simulink model "STDiscovery"  (R2017b)
settings: Solver=FixedStepAuto  StartTime=0.0  StopTime=0.01  FixedStep=Abtastzeit  RelTol=1e-3
PreLoadFcn:
  | waijung.modelPreload; % Required for working with Waijung Blockset. Do not remove.
model workspace (MAT data in the model file):
  Abtastzeit = 0.01
  Servo_IN_min = 0.894
  SimulationDutyCycle = 27
undefined symbols (not defined in the file): HSEOSC, Link, LQFP176, ST, Statusbits, Steuerbits, STM32F417IG
libraries: simulink x17, stm32f4_io_lib x16, simulink_extras x8, stm32f4_adc_lib x7, powerlib_meascontrol x4, stm32f4_device_config_lib x1
(part 2 of 4)

== system STDiscovery/MomentangeschwindigkeitEinlesen ==
  note: Umrechnung Hz nach m/s
  Data Store Write : DataStoreWrite  DataStoreName=MomentanGeschwindigkeit_MeterProSekunde
  Fernbediehnung Motor : S-Function  FunctionName=stm32f4_pwm_capture  Parameters=conf,inputporttype,inputportwidth,outputporttype,outputportwidth,optionstring,sampletime,blockid  SFunctionDeploymentMode=off  EnableBusSupport=off  mask(stm32f4_pwm_capture){conf=Capture, timer=3, lasttimer=3, pin=C7, pintype=Pull Up, edge=Rising, datatype=single, portpinstr=0, sampletime=Abtastzeit, blockid=MomentangeschwindigkeitEinlesenFernbediehnungMotor, inputporttype=[], inputportwidth=[], inputportlabel={}, outputporttype=[3 1 1 1], outputportwidth=[], outputportlabel={'READY','+Width (sec)','+Duty (%)','Frequency (Hz)'}, compat=0, optionstring=["3","1","C","7","2","16","Rising","UP","float"]}
      mask prompts: conf "Configuration"; lasttimer "Last Timer"; pin "Capture Pin"; pintype "Capture Pin Type (Pull-Up/Pull-Down)"; edge "Capture Edge"; datatype "Output data type"; portpinstr "Port Pin String"; sampletime "Sample time (sec)"; blockid "Block ID"; inputporttype "Input Port Type"; inputportwidth "Input Port Width"; inputportlabel "Input Port Label"; outputporttype "Output Port Type"; outputportwidth "Output Port Width"; outputportlabel "Output port label"; compat "Compatibility (Reserved for future use)"; optionstring "String(s) to be passed to TLC"
      mask help:
      | Capture Edge:
      |  Rising - PWM period start from rising edge of pulse N to rising edge of pulse N+1
      |  Falling - PWM period start from falling edge of pulse N to falling edge of pulse N+1
      | Capture data type:
      |  Capture data type, selectable to double or single.
      |
      | Output:
      |  READY - indicate the status of capture, a non-zero value indicate data is ready.
      |  +Width - positive pulse width, in unit of second.
      |  +Duty - positive duty cycle, 0 to 100%
      |  Frequency - signal frequency in unit of Hz
      |
      | Note: caprure period should not longer than 1 second (Maximum limit is 3 seconds)
      mask init:
      | stm32f4_pwm_capture_callback('init');
      mask Help: web(fullfile(waijungdocroot,'stm32f4_pwm_capture.htm'), '-browser')
      mask TypeOptions conf: Capture
      mask Callback conf: stm32f4_pwm_capture_callback('conf');
      mask TypeOptions timer: 1 | 2 | 3 | 4 | 5 | 8
      mask Callback timer: stm32f4_pwm_capture_callback('timer');
      mask TypeOptions pin: Not used | A6 | B4 | C6 | A7 | B5 | C7 | B0 | C8 | B1 | C9
      mask TypeOptions pintype: None | Pull Up | Pull Down
      mask TypeOptions edge: Rising | Falling
      mask TypeOptions datatype: double | single
      mask Callback sampletime: stm32f4_pwm_capture_callback('sampletime');
      mask Callback blockid: stm32f4_pwm_capture_callback('blockid');
      mask Display: text(0.05, 0.5, 'Timer: 3 (16 bit)\nInput Pin: C7\nEdge: Rising\nTs (sec): -1','ver','middle','hor','left'); port_label('output', 1,'READY'); port_label('output', 2,'+Width (sec)'); port_label('output', 3,'+Duty (%)'); port_label('output', 4,'Frequency (Hz)');
  MATLAB Function : MATLAB Function  TreatAsAtomicUnit=on
  Saturation : Saturate  UpperLimit=10  LowerLimit=0
  Terminator : Terminator
  Terminator1 : Terminator
  Terminator2 : Terminator
  wires:
  MATLAB Function/1(y) -> Saturation/1
  Saturation/1 -> Data Store Write/1
  Fernbediehnung Motor/4 -> MATLAB Function/1(x)
  Fernbediehnung Motor/1 -> Terminator/1
  Fernbediehnung Motor/2 -> Terminator1/1
  Fernbediehnung Motor/3 -> Terminator2/1

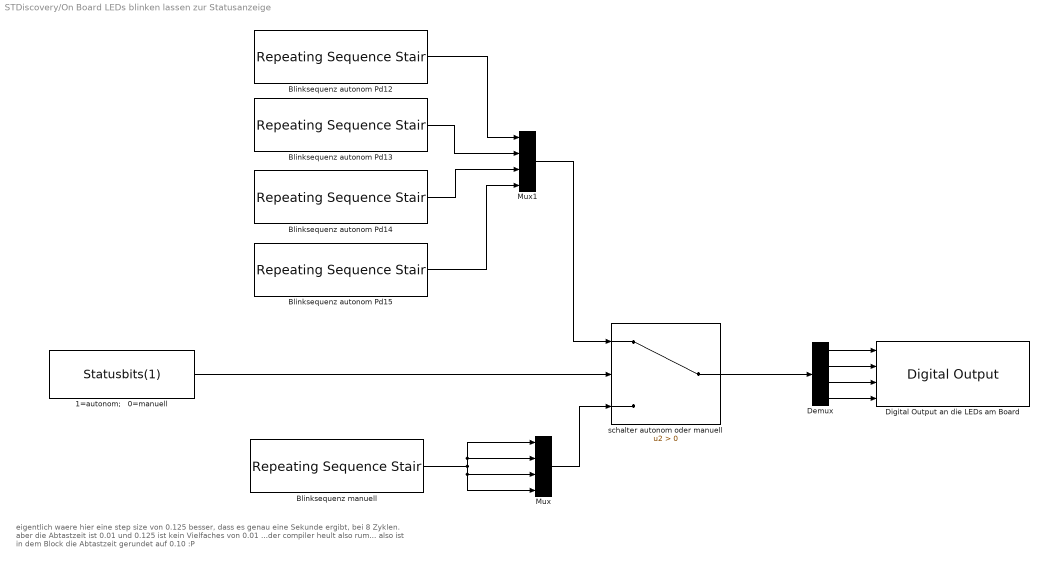
== system STDiscovery/On Board LEDs blinken lassen zur Statusanzeige ==
  note: eigentlich waere hier eine step size von 0.125 besser, dass es genau eine Sekunde ergibt, bei 8 Zyklen.
      | aber die Abtastzeit ist 0.01 und 0.125 ist kein Vielfaches von 0.01 ...der compiler heult also rum...
      | also ist in dem Block die Abtastzeit gerundet auf 0.10 :P
  1=autonom;   0=manuell : DataStoreRead  DataStoreName=Statusbits  DataStoreElements=Statusbits(1)
  Blinksequenz autonom Pd12 : simulink/Sources/Repeating Sequence Stair  OutValues=[1 0 0 0].'  tsamp=0.1  OutMin=[]  OutMax=[]  OutDataTypeStr=double  OutputDataTypeScalingMode=double  OutDataType=fixdt(0,8)  ConRadixGroup=Best Precision: Vector-wise  OutScaling=2^-12
  Blinksequenz autonom Pd13 : simulink/Sources/Repeating Sequence Stair  OutValues=[0 1 0 0 ].'  tsamp=0.1  OutMin=[]  OutMax=[]  OutDataTypeStr=double  OutputDataTypeScalingMode=double  OutDataType=fixdt(0,8)  ConRadixGroup=Best Precision: Vector-wise  OutScaling=2^-12
  Blinksequenz autonom Pd14 : simulink/Sources/Repeating Sequence Stair  OutValues=[0 0 1 0].'  tsamp=0.1  OutMin=[]  OutMax=[]  OutDataTypeStr=double  OutputDataTypeScalingMode=double  OutDataType=fixdt(0,8)  ConRadixGroup=Best Precision: Vector-wise  OutScaling=2^-12
  Blinksequenz autonom Pd15 : simulink/Sources/Repeating Sequence Stair  OutValues="[0 0 0 1  ].'"  tsamp=0.1  OutMin=[]  OutMax=[]  OutDataTypeStr=double  OutputDataTypeScalingMode=double  OutDataType=fixdt(0,8)  ConRadixGroup=Best Precision: Vector-wise  OutScaling=2^-12
  Blinksequenz manuell : simulink/Sources/Repeating Sequence Stair  OutValues=[1 0 1 0 0 0 0 0 0 0].'  tsamp=0.1  OutMin=[]  OutMax=[]  OutDataTypeStr=double  OutputDataTypeScalingMode=double  OutDataType=fixdt(0,8)  ConRadixGroup=Best Precision: Vector-wise  OutScaling=2^-12
  Demux : Demux
  Digital Output an die LEDs am Board : stm32f4_io_lib/Digital Output  use_bitband=on  port=D  speed=100  porttype=Push Pull  porttypestr=PP  use_pin0=off  use_pin1=off  use_pin2=off  use_pin3=off  use_pin4=off  use_pin5=off  use_pin6=off  use_pin7=off  use_pin8=off  use_pin9=off  use_pin10=off  use_pin11=off  use_pin12=on  use_pin13=on  use_pin14=on  use_pin15=on  pinstr=GPIO_Pin_12 | GPIO_Pin_13 | GPIO_Pin_14 | GPIO_Pin_15  usedpinarray="[0  0  0  0  0  0  0  0  0  0  0  0  1  1  1  1]"  bitbandingstr=|  sampletime=-1  sampletimestr=-1  blockid=OnBoardLEDsblinkenlassenzurStatusanzeigeDigitalOutputandieLEDsamBoard  enablecustomportlabel=off  globalinit=off  cinputportlabel=In1, In2  coutputportlabel=0
      | #define OnBoardLEDsblinkenlassenzurStatusanzeigeDigitalOutputandieLEDsamBoard_D12 Peripheral_BB(GPIOD->ODR, 12)  /* Output pin */
      | #define OnBoardLEDsblinkenlassenzurStatusanzeigeDigitalOutputandieLEDsamBoard_D13 Peripheral_BB(GPIOD->ODR, 13)  /* Output pin */
      | #define OnBoardLEDsblinkenlassenzurStatusanzeigeDigitalOutputandieLEDsamBoard_D14 Peripheral_BB(GPIOD->ODR, 14)  /* Output pin */
      | #define OnBoardLEDsblinkenlassenzurStatusanzeigeDigitalOutputandieLEDsamBoard_D15 Peripheral_BB(GPIOD->ODR, 15)  /* Output pin */
      settings: SourceProductName=Waijung Blockset
  Mux : Mux
  Mux1 : Mux
  schalter autonom oder manuell : Switch  Criteria=u2 > Threshold
  wires:
  1=autonom;   0=manuell/1 -> schalter autonom oder manuell/2
  Demux/1 -> Digital Output an die LEDs am Board/1
  Demux/2 -> Digital Output an die LEDs am Board/2
  Demux/3 -> Digital Output an die LEDs am Board/3
  Demux/4 -> Digital Output an die LEDs am Board/4
  schalter autonom oder manuell/1 -> Demux/1
  Mux/1 -> schalter autonom oder manuell/3
  Blinksequenz manuell/1 -> Mux/2, Mux/1, Mux/4, Mux/3
  Blinksequenz autonom Pd12/1 -> Mux1/1
  Blinksequenz autonom Pd13/1 -> Mux1/2
  Blinksequenz autonom Pd14/1 -> Mux1/3
  Blinksequenz autonom Pd15/1 -> Mux1/4
  Mux1/1 -> schalter autonom oder manuell/1

== system STDiscovery/Power Distribution Unit ==
  note: Sicherungen
  Sicherung Akku : Subsystem
  Sicherung Jetson : Subsystem
  Sicherung Motor : Subsystem
  Sicherung Reciever : Subsystem
  Sicherung ST : Subsystem
  Sicherung Servo : Subsystem
  Sicherung Spare : Subsystem

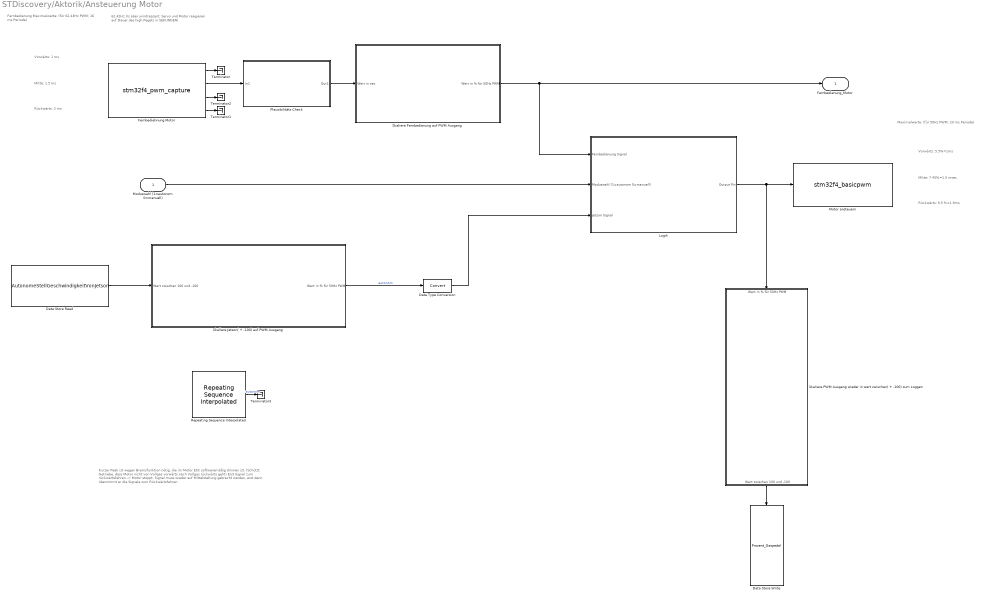
== system STDiscovery/Aktorik/Ansteuerung Motor ==
  note: Kurzer Peak ist wegen Bremsfunktion nötig, die im Motor ESC softwaremäßig drinnen ist.
      | (Schützt Getriebe, dass Motor nicht von Vollgas vorwärts nach Vollgas rückwärts geht)
      | Erst Signal zum rückwärtsfahren.-> Motor stoppt, Signal muss wieder auf Mittelstellung
      | gebracht werden, erst dann übernimmt er die Signale zum Rückwärtsfahren
  note: Vorwärts:
      | 1 ms
  note: Mitte:
      | 1.5 ms
  note: Rückwärts:
      | 2 ms
  note: 62.42Hz (Is aber unintressant,
      | Servo und Motor reagieren
      | auf Dauer des high Pegels
      | in SEKUNDEN)
  note: Rückwärts:
      | 9.5 %=1.9ms
  note: Vorwärts:
      | 5.5%=1ms
  note: Mitte:
      | 7.45%=1.5 msec
  note: Maximalwerte:
      | (für 50Hz PWM; 20 ms Periode)
  note: Fernbedienung Maximalwerte:
      | (für 62.43Hz PWM; 16 ms Periode)
  Moduswahl (1=autonom 0=manuell) : Inport
  Data Store Read : DataStoreRead  DataStoreName=AutonomeStellGeschwindigkeitVonJetson
  Data Store Write : DataStoreWrite  DataStoreName=Prozent_Gaspedal
  Data Type Conversion : DataTypeConversion
  Fernbediehnung Motor : S-Function  FunctionName=stm32f4_pwm_capture  Parameters=conf,inputporttype,inputportwidth,outputporttype,outputportwidth,optionstring,sampletime,blockid  SFunctionDeploymentMode=off  EnableBusSupport=off  mask(stm32f4_pwm_capture){conf=Capture, timer=2, lasttimer=2, pin=A15, pintype=Pull Up, edge=Rising, datatype=single, portpinstr=0, sampletime=Abtastzeit, blockid=AktorikAnsteuerungMotorFernbediehnungMotor, inputporttype=[], inputportwidth=[], inputportlabel={}, outputporttype=[3 1 1 1], outputportwidth=[], outputportlabel={'READY','+Width (sec)','+Duty (%)','Frequency (Hz)'}, compat=0, optionstring=["2","1","A","15","1","32","Rising","UP","float"]}
      mask prompts: conf "Configuration"; lasttimer "Last Timer"; pin "Capture Pin"; pintype "Capture Pin Type (Pull-Up/Pull-Down)"; edge "Capture Edge"; datatype "Output data type"; portpinstr "Port Pin String"; sampletime "Sample time (sec)"; blockid "Block ID"; inputporttype "Input Port Type"; inputportwidth "Input Port Width"; inputportlabel "Input Port Label"; outputporttype "Output Port Type"; outputportwidth "Output Port Width"; outputportlabel "Output port label"; compat "Compatibility (Reserved for future use)"; optionstring "String(s) to be passed to TLC"
      mask help:
      | Capture Edge:
      |  Rising - PWM period start from rising edge of pulse N to rising edge of pulse N+1
      |  Falling - PWM period start from falling edge of pulse N to falling edge of pulse N+1
      | Capture data type:
      |  Capture data type, selectable to double or single.
      |
      | Output:
      |  READY - indicate the status of capture, a non-zero value indicate data is ready.
      |  +Width - positive pulse width, in unit of second.
      |  +Duty - positive duty cycle, 0 to 100%
      |  Frequency - signal frequency in unit of Hz
      |
      | Note: caprure period should not longer than 1 second (Maximum limit is 3 seconds)
      mask init:
      | stm32f4_pwm_capture_callback('init');
      mask Help: web(fullfile(waijungdocroot,'stm32f4_pwm_capture.htm'), '-browser')
      mask TypeOptions conf: Capture
      mask Callback conf: stm32f4_pwm_capture_callback('conf');
      mask TypeOptions timer: 1 | 2 | 3 | 4 | 5 | 8
      mask Callback timer: stm32f4_pwm_capture_callback('timer');
      mask TypeOptions pin: Not used | A0 | A5 | A15 | A1 | B3 | A2 | B10 | A3 | B11
      mask TypeOptions pintype: None | Pull Up | Pull Down
      mask TypeOptions edge: Rising | Falling
      mask TypeOptions datatype: double | single
      mask Callback sampletime: stm32f4_pwm_capture_callback('sampletime');
      mask Callback blockid: stm32f4_pwm_capture_callback('blockid');
      mask Display: text(0.05, 0.5, 'Timer: 2 (32 bit)\nInput Pin: A15\nEdge: Rising\nTs (sec): -1','ver','middle','hor','left'); port_label('output', 1,'READY'); port_label('output', 2,'+Width (sec)'); port_label('output', 3,'+Duty (%)'); port_label('output', 4,'Frequency (Hz)');
  "Logik " : Subsystem
  Motor ansteuern : S-Function  FunctionName=stm32f4_basicpwm  Parameters=timer,pwmperiod,ch1pin,ch2pin,ch3pin,ch4pin,sampletime,sampletimestr,blockid,apb,portstr,pinstr,pinmat,timarr,timprescale,chmat,polaritystr  SFunctionDeploymentMode=off  EnableBusSupport=off  mask(stm32f4_basicpwm){timer=10, pwmperiod=0.02, polarity=Active High, polaritystr=TIM_OCPolarity_High, ch1pin=B8, ch2pin=Not available - Do not use, ch3pin=Not available - Do not use, ch4pin=Not available - Do not use, sampletime=Abtastzeit, sampletimestr=-1, blockid=AktorikAnsteuerungMotorMotoransteuern, portpinstr=B8,,,, enablecustomportlabel=off, cinputportlabel=In1, In2, In3, In4, coutputportlabel=0, apb=2, portstr=["B"], pinstr=["GPIO_Pin_8"], pinmat=[1 8], timarr=64614, timprescale=51, chmat=[1]}
      mask prompts: pwmperiod "PWM Period (seconds)"; ch1pin "Channel 1"; ch2pin "Channel 2"; ch3pin "Channel 3"; ch4pin "Channel 4"; sampletime "Sample time (sec)"; sampletimestr "Compiled sample time (sec) in string"; portpinstr "Port pin string"; enablecustomportlabel "Enable custom port labels"; cinputportlabel "Custom input port labels (Ex. In1, In2, In3)"; coutputportlabel "Custom output port labels (Ex. Out1, Out2, Out3)"; portstr "Port string"; pinstr "Pin string"; pinmat "Pin matrix"; timarr "Timer ARR"; timprescale "Timer PRESCALE"; chmat "Channel order"
      mask help:
      | This block implements basic Edge-aligned Pulse Width Modulation (PWM) generation.
      | All timers are 16-bit. The PWM period is fixed (per timer).
      mask init:
      | stm32f4_basicpwm_callback('init');
      mask Help: web(fullfile(waijungdocroot,'stm32f4_basicpwm.htm'),'-browser')
      mask TypeOptions timer: 1 | 2 | 3 | 4 | 5 | 8 | 9 | 10 | 11 | 12 | 13 | 14
      mask Callback timer: stm32f4_basicpwm_callback('timer');
      mask Callback pwmperiod: stm32f4_basicpwm_callback('pwmperiod');
      mask TypeOptions polarity: Active High | Active Low
      mask Callback polarity: stm32f4_basicpwm_callback('polarity');
      mask TypeOptions ch1pin: Not available - Do not use | B8
      mask Callback ch1pin: stm32f4_basicpwm_callback('ch1pin');
      mask TypeOptions ch2pin: Not available - Do not use
      mask Callback ch2pin: stm32f4_basicpwm_callback('ch2pin');
      mask TypeOptions ch3pin: Not available - Do not use
      mask Callback ch3pin: stm32f4_basicpwm_callback('ch3pin');
      mask TypeOptions ch4pin: Not available - Do not use
      mask Callback ch4pin: stm32f4_basicpwm_callback('ch4pin');
      mask Callback sampletime: stm32f4_basicpwm_callback('sampletime');
      mask Callback sampletimestr: stm32f4_basicpwm_callback('sampletimestr');
      mask Callback blockid: stm32f4_basicpwm_callback('blockid');
      mask Callback enablecustomportlabel: stm32f4_basicpwm_callback('enablecustomportlabel');
      mask Display: text(0.95, 0.5, 'Timer: 10\nPolarity: Active High\nPeriod (sec) 0.02\nTs (sec): -1','ver','middle','hor','right');port_label('input', 1,'CH1 (B8)')
  Plausibilitäts Check : Subsystem
  Repeating Sequence Interpolated : simulink/Sources/Repeating Sequence Interpolated  OutValues=[7.45 5.5 7.45 8 7.45 9.5 7.45]  TimeValues=[0 4 8 8.3 8.6 12.6 16.6 ].'  LookUpMeth=Interpolation-Use End Values  tsamp=0.01  OutMin=[]  OutMax=[]  OutDataTypeStr=double  OutputDataTypeScalingMode=double  OutDataType=fixdt(0,8)  OutScaling=2^-10
  Skaliere Fernbedienung auf PWM Ausgang : Subsystem
  Skaliere Jetson( + -100) auf PWM Ausgang : Subsystem
  "Skaliere PWM Ausgang wieder in wert zwischen( + -100) zum Loggen " : Subsystem
  Terminator{,1..3} (4 alike) : Terminator
  Fernbedienung_Motor : Outport
  wires:
  Fernbediehnung Motor/3 -> Terminator2/1
  Fernbediehnung Motor/1 -> Terminator/1
  Fernbediehnung Motor/4 -> Terminator1/1
  Fernbediehnung Motor/2 -> Plausibilitäts Check/1(In1)
  "Logik "/1(Output Pin) -> "Skaliere PWM Ausgang wieder in wert zwischen( + -100) zum Loggen "/1(Wert in % für 50Hz PWM), Motor ansteuern/1
  Skaliere Jetson( + -100) auf PWM Ausgang/1(Wert in % für 50Hz PWM) -> Data Type Conversion/1  "autonom"
  Plausibilitäts Check/1(Out1) -> Skaliere Fernbedienung auf PWM Ausgang/1(Wert in sec)
  Moduswahl (1=autonom 0=manuell)/1 -> "Logik "/2(Moduswahl (1=autonom 0=manuell))
  Skaliere Fernbedienung auf PWM Ausgang/1(Wert in % für 50Hz PWM) -> "Logik "/1(Fernbedienung Signal), Fernbedienung_Motor/1
  Data Store Read/1 -> Skaliere Jetson( + -100) auf PWM Ausgang/1(Wert zwischen 100 und -100)
  Data Type Conversion/1 -> "Logik "/3(Jetson Signal)
  Repeating Sequence Interpolated/1 -> Terminator3/1  "autonom"
  "Skaliere PWM Ausgang wieder in wert zwischen( + -100) zum Loggen "/1("Wert zwischen 100 und -100 ") -> Data Store Write/1

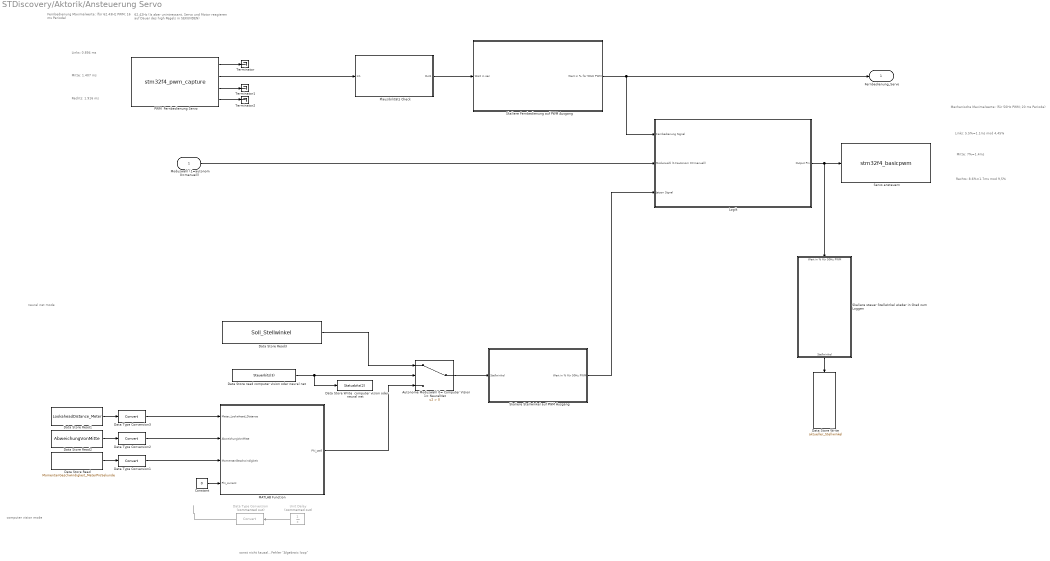
== system STDiscovery/Aktorik/Ansteuerung Servo ==
  note: neural net mode
  note: sonst nicht kausal...Fehler "Algebraic loop"
  note: Mechanische Maximalwerte:
      | (für 50Hz PWM; 20 ms Periode)
  note: 62.42Hz (Is aber unintressant,
      | Servo und Motor reagieren
      | auf Dauer des high Pegels
      | in SEKUNDEN)
  note: Mitte:
      | 1.407 ms
  note: Links:
      | 0.894 ms
  note: Rechts:
      | 1.916 ms
  note: Links:
      | 5.5%=1.1ms mod 4,45%
  note: Mitte:
      | 7%=1.4ms
  note: Rechts:
      | 8.6%=1.7ms mod 9,5%
  note: Fernbedienung Maximalwerte:
      | (für 62.43Hz PWM; 16 ms Periode)
  note: computer vision mode
  Moduswahl (1=autonom 0=manuell) : Inport
  Autonome Moduswahl 0= Computer Vision 1= NeuralNet : Switch  Criteria=u2 > Threshold
  Constant : Constant  Value=0
  Data Store Read : DataStoreRead  DataStoreName=MomentanGeschwindigkeit_MeterProSekunde
  Data Store Read1 : DataStoreRead  DataStoreName=LookaheadDistance_Meter
  Data Store Read2 : DataStoreRead  DataStoreName=AbweichungVonMitte
  Data Store Read3 : DataStoreRead  DataStoreName=Soll_Stellwinkel
  Data Store Write : DataStoreWrite  DataStoreName=aktueller_Stellwinkel
  Data Store Write  computer vision oder neural net : DataStoreWrite  DataStoreName=Statusbits  DataStoreElements=Statusbits(2)
  Data Store read computer vision oder neural net : DataStoreRead  DataStoreName=Steuerbits  DataStoreElements=Steuerbits(3)
  Data Type Conversion : DataTypeConversion  Commented=on
  Data Type Conversion1 : DataTypeConversion
  Data Type Conversion2 : DataTypeConversion
  Data Type Conversion3 : DataTypeConversion
  "Logik " : Subsystem
  MATLAB Function : MATLAB Function  TreatAsAtomicUnit=on
  PWM  Fernbedienung Servo : S-Function  FunctionName=stm32f4_pwm_capture  Parameters=conf,inputporttype,inputportwidth,outputporttype,outputportwidth,optionstring,sampletime,blockid  SFunctionDeploymentMode=off  EnableBusSupport=off  mask(stm32f4_pwm_capture){conf=Capture, timer=1, lasttimer=1, pin=A8, pintype=Pull Up, edge=Rising, datatype=single, portpinstr=0, sampletime=Abtastzeit, blockid=AktorikAnsteuerungServoPWMFernbedienungServo, inputporttype=[], inputportwidth=[], inputportlabel={}, outputporttype=[3 1 1 1], outputportwidth=[], outputportlabel={'READY','+Width (sec)','+Duty (%)','Frequency (Hz)'}, compat=0, optionstring=["1","2","A","8","1","16","Rising","UP","float"]}
      mask prompts: conf "Configuration"; lasttimer "Last Timer"; pin "Capture Pin"; pintype "Capture Pin Type (Pull-Up/Pull-Down)"; edge "Capture Edge"; datatype "Output data type"; portpinstr "Port Pin String"; sampletime "Sample time (sec)"; blockid "Block ID"; inputporttype "Input Port Type"; inputportwidth "Input Port Width"; inputportlabel "Input Port Label"; outputporttype "Output Port Type"; outputportwidth "Output Port Width"; outputportlabel "Output port label"; compat "Compatibility (Reserved for future use)"; optionstring "String(s) to be passed to TLC"
      mask help:
      | Capture Edge:
      |  Rising - PWM period start from rising edge of pulse N to rising edge of pulse N+1
      |  Falling - PWM period start from falling edge of pulse N to falling edge of pulse N+1
      | Capture data type:
      |  Capture data type, selectable to double or single.
      |
      | Output:
      |  READY - indicate the status of capture, a non-zero value indicate data is ready.
      |  +Width - positive pulse width, in unit of second.
      |  +Duty - positive duty cycle, 0 to 100%
      |  Frequency - signal frequency in unit of Hz
      |
      | Note: caprure period should not longer than 1 second (Maximum limit is 3 seconds)
      mask init:
      | stm32f4_pwm_capture_callback('init');
      mask Help: web(fullfile(waijungdocroot,'stm32f4_pwm_capture.htm'), '-browser')
      mask TypeOptions conf: Capture
      mask Callback conf: stm32f4_pwm_capture_callback('conf');
      mask TypeOptions timer: 1 | 2 | 3 | 4 | 5 | 8
      mask Callback timer: stm32f4_pwm_capture_callback('timer');
      mask TypeOptions pin: Not used | A8 | E9 | A9 | E11 | A10 | E13 | A11 | E14
      mask TypeOptions pintype: None | Pull Up | Pull Down
      mask TypeOptions edge: Rising | Falling
      mask TypeOptions datatype: double | single
      mask Callback sampletime: stm32f4_pwm_capture_callback('sampletime');
      mask Callback blockid: stm32f4_pwm_capture_callback('blockid');
      mask Display: text(0.05, 0.5, 'Timer: 1 (16 bit)\nInput Pin: A8\nEdge: Rising\nTs (sec): -1','ver','middle','hor','left'); port_label('output', 1,'READY'); port_label('output', 2,'+Width (sec)'); port_label('output', 3,'+Duty (%)'); port_label('output', 4,'Frequency (Hz)');
  Plausibilitäts Check : Subsystem
  Servo ansteuern : S-Function  FunctionName=stm32f4_basicpwm  Parameters=timer,pwmperiod,ch1pin,ch2pin,ch3pin,ch4pin,sampletime,sampletimestr,blockid,apb,portstr,pinstr,pinmat,timarr,timprescale,chmat,polaritystr  SFunctionDeploymentMode=off  EnableBusSupport=off  mask(stm32f4_basicpwm){timer=9, pwmperiod=0.02, polarity=Active High, polaritystr=TIM_OCPolarity_High, ch1pin=E5, ch2pin=Not available - Do not use, ch3pin=Not available - Do not use, ch4pin=Not available - Do not use, sampletime=Abtastzeit, sampletimestr=-1, blockid=AktorikAnsteuerungServoServoansteuern, portpinstr=E5,,,, enablecustomportlabel=off, cinputportlabel=In1, In2, In3, In4, coutputportlabel=0, apb=2, portstr=["E"], pinstr=["GPIO_Pin_5"], pinmat=[1 5], timarr=64614, timprescale=51, chmat=[1]}
      mask prompts: pwmperiod "PWM Period (seconds)"; ch1pin "Channel 1"; ch2pin "Channel 2"; ch3pin "Channel 3"; ch4pin "Channel 4"; sampletime "Sample time (sec)"; sampletimestr "Compiled sample time (sec) in string"; portpinstr "Port pin string"; enablecustomportlabel "Enable custom port labels"; cinputportlabel "Custom input port labels (Ex. In1, In2, In3)"; coutputportlabel "Custom output port labels (Ex. Out1, Out2, Out3)"; portstr "Port string"; pinstr "Pin string"; pinmat "Pin matrix"; timarr "Timer ARR"; timprescale "Timer PRESCALE"; chmat "Channel order"
      mask help:
      | This block implements basic Edge-aligned Pulse Width Modulation (PWM) generation.
      | All timers are 16-bit. The PWM period is fixed (per timer).
      mask init:
      | stm32f4_basicpwm_callback('init');
      mask Help: web(fullfile(waijungdocroot,'stm32f4_basicpwm.htm'),'-browser')
      mask TypeOptions timer: 1 | 2 | 3 | 4 | 5 | 8 | 9 | 10 | 11 | 12 | 13 | 14
      mask Callback timer: stm32f4_basicpwm_callback('timer');
      mask Callback pwmperiod: stm32f4_basicpwm_callback('pwmperiod');
      mask TypeOptions polarity: Active High | Active Low
      mask Callback polarity: stm32f4_basicpwm_callback('polarity');
      mask TypeOptions ch1pin: Not available - Do not use | A2 | E5
      mask Callback ch1pin: stm32f4_basicpwm_callback('ch1pin');
      mask TypeOptions ch2pin: Not available - Do not use | A3 | E6
      mask Callback ch2pin: stm32f4_basicpwm_callback('ch2pin');
      mask TypeOptions ch3pin: Not available - Do not use
      mask Callback ch3pin: stm32f4_basicpwm_callback('ch3pin');
      mask TypeOptions ch4pin: Not available - Do not use
      mask Callback ch4pin: stm32f4_basicpwm_callback('ch4pin');
      mask Callback sampletime: stm32f4_basicpwm_callback('sampletime');
      mask Callback sampletimestr: stm32f4_basicpwm_callback('sampletimestr');
      mask Callback blockid: stm32f4_basicpwm_callback('blockid');
      mask Callback enablecustomportlabel: stm32f4_basicpwm_callback('enablecustomportlabel');
      mask Display: text(0.95, 0.5, 'Timer: 9\nPolarity: Active High\nPeriod (sec) 0.02\nTs (sec): -1','ver','middle','hor','right');port_label('input', 1,'CH1 (E5)')
  Skaliere Fernbedienung auf PWM Ausgang : Subsystem
  Skaliere Stellwinkel auf PWM Ausgang : Subsystem
  Skaliere steuer Stellwinkel wieder in Grad zum Loggen : Subsystem
  Terminator : Terminator
  Terminator1 : Terminator
  Terminator2 : Terminator
  Unit Delay : UnitDelay  Commented=on  SampleTime=-1
  Fernbedienung_Servo : Outport
  wires:
  Skaliere Stellwinkel auf PWM Ausgang/1(Wert in % für 50Hz PWM) -> "Logik "/3(Jetson Signal)
  PWM  Fernbedienung Servo/1 -> Terminator/1
  PWM  Fernbedienung Servo/3 -> Terminator1/1
  PWM  Fernbedienung Servo/4 -> Terminator2/1
  PWM  Fernbedienung Servo/2 -> Plausibilitäts Check/1(In1)
  Skaliere Fernbedienung auf PWM Ausgang/1(Wert in % für 50Hz PWM) -> Fernbedienung_Servo/1, "Logik "/1(Fernbedienung Signal)
  Plausibilitäts Check/1(Out1) -> Skaliere Fernbedienung auf PWM Ausgang/1(Wert in sec)
  "Logik "/1(Output Pin) -> Servo ansteuern/1, Skaliere steuer Stellwinkel wieder in Grad zum Loggen/1(Wert in % für 50Hz PWM)
  Moduswahl (1=autonom 0=manuell)/1 -> "Logik "/2(Moduswahl (1=autonom 0=manuell))
  Data Store Read1/1 -> Data Type Conversion3/1
  Data Store Read/1 -> Data Type Conversion1/1
  Data Store Read2/1 -> Data Type Conversion2/1
  Data Type Conversion/1 -> ?
  MATLAB Function/1(Phi_stell) -> Autonome Moduswahl 0= Computer Vision 1= NeuralNet/3
  Unit Delay/1 -> Data Type Conversion/1
  Data Type Conversion1/1 -> MATLAB Function/3(MomentanGeschwindigkeit)
  Data Type Conversion2/1 -> MATLAB Function/2(AbweichungVonMitte)
  Data Type Conversion3/1 -> MATLAB Function/1(Meter_Lookahead_Distance)
  Constant/1 -> MATLAB Function/4(Phi_current)
  Skaliere steuer Stellwinkel wieder in Grad zum Loggen/1(Stellwinkel) -> Data Store Write/1
  Autonome Moduswahl 0= Computer Vision 1= NeuralNet/1 -> Skaliere Stellwinkel auf PWM Ausgang/1(Stellwinkel)
  Data Store Read3/1 -> Autonome Moduswahl 0= Computer Vision 1= NeuralNet/1
  Data Store read computer vision oder neural net/1 -> Data Store Write  computer vision oder neural net/1, Autonome Moduswahl 0= Computer Vision 1= NeuralNet/2

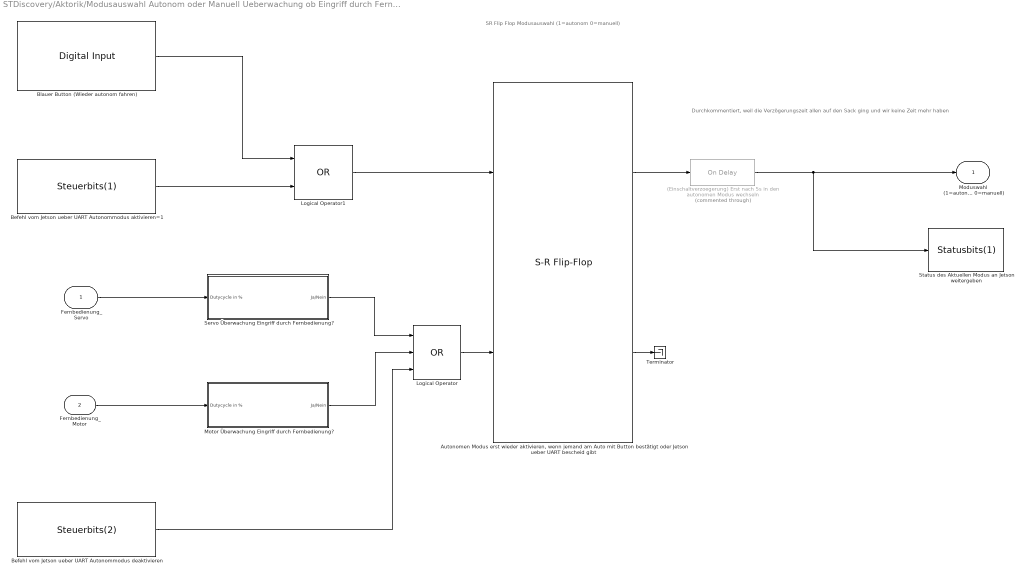
== system STDiscovery/Aktorik/Modusauswahl Autonom oder Manuell Ueberwachung ob Eingriff durch Fernbedienung ==
  note: Durchkommentiert, weil die Verzögerungszeit allen auf den Sack ging
      | und wir keine Zeit mehr haben
  note: SR Flip Flop Modusauswahl
      | (1=autonom 0=manuell)
  Fernbedienung_Servo : Inport
  Fernbedienung_Motor : Inport  Port=2
  (Einschaltverzoegerung) Erst nach 5s in den autonomen Modus wechseln : powerlib_meascontrol/Logic/On Delay  Commented=through  DelayType=On delay  delay=5  ic=1  Ts=0
      settings: SourceProductName=Simscape Power Systems
  "Autonomen Modus erst wieder aktivieren, wenn jemand am Auto mit Button bestätigt oder Jetson ueber UART bescheid gibt" : simulink_extras/Flip Flops/S-R Flip-Flop  initial_condition=0
  Befehl vom Jetson ueber UART Autonommodus aktivieren=1 : DataStoreRead  DataStoreName=Steuerbits  DataStoreElements=Steuerbits(1)
  Befehl vom Jetson ueber UART Autonommodus deaktivieren : DataStoreRead  DataStoreName=Steuerbits  DataStoreElements=Steuerbits(2)
  Blauer Button (Wieder autonom fahren) : stm32f4_io_lib/Digital Input  port=A  speed=100  porttype=None  porttypestr=NOPULL  use_pin0=on  use_pin1=off  use_pin2=off  use_pin3=off  use_pin4=off  use_pin5=off  use_pin6=off  use_pin7=off  use_pin8=off  use_pin9=off  use_pin10=off  use_pin11=off  use_pin12=off  use_pin13=off  use_pin14=off  use_pin15=off  pinstr=GPIO_Pin_0  usedpinarray="[1  0  0  0  0  0  0  0  0  0  0  0  0  0  0  0]"  bitbandingstr="#define AktorikModusauswahlAutonomoderManuellUeberwachungobEingriffdurchFernbedienungBlauerButtonWiederautonomfahren_A0 Peripheral_BB(GPIOA->IDR, 0)  /* Output pin */"  sampletime=0.1  sampletimestr=-1  blockid=AktorikModusauswahlAutonomoderManuellUeberwachungobEingriffdurchFernbedienungBlauerButtonWiederautonomfahren  enablecustomportlabel=off  glabalinit=off  cinputportlabel=In1, In2  coutputportlabel=Out1, Out2
      settings: SourceProductName=Waijung Blockset
  Logical Operator : Logic  Operator=OR  Inputs=3  AllPortsSameDT=off  OutDataTypeStr=boolean
  Logical Operator1 : Logic  Operator=OR  AllPortsSameDT=off  OutDataTypeStr=boolean
  Motor Überwachung Eingriff durch Fernbedienung? : Subsystem
  Servo Überwachung Eingriff durch Fernbedienung? : Subsystem
  Status des Aktuellen Modus an Jetson weitergeben : DataStoreWrite  DataStoreName=Statusbits  DataStoreElements=Statusbits(1)
  Terminator : Terminator
  Moduswahl (1=autonom 0=manuell) : Outport
  wires:
  "Autonomen Modus erst wieder aktivieren, wenn jemand am Auto mit Button bestätigt oder Jetson ueber UART bescheid gibt"/1 -> (Einschaltverzoegerung) Erst nach 5s in den autonomen Modus wechseln/1
  (Einschaltverzoegerung) Erst nach 5s in den autonomen Modus wechseln/1 -> Status des Aktuellen Modus an Jetson weitergeben/1, Moduswahl (1=autonom 0=manuell)/1
  "Autonomen Modus erst wieder aktivieren, wenn jemand am Auto mit Button bestätigt oder Jetson ueber UART bescheid gibt"/2 -> Terminator/1
  Befehl vom Jetson ueber UART Autonommodus aktivieren=1/1 -> Logical Operator1/2
  Blauer Button (Wieder autonom fahren)/1 -> Logical Operator1/1
  Fernbedienung_Motor/1 -> Motor Überwachung Eingriff durch Fernbedienung?/1(Dutycycle in %)
  Fernbedienung_Servo/1 -> Servo Überwachung Eingriff durch Fernbedienung?/1(Dutycycle in %)
  Servo Überwachung Eingriff durch Fernbedienung?/1(Ja/Nein) -> Logical Operator/1
  Motor Überwachung Eingriff durch Fernbedienung?/1(Ja/Nein) -> Logical Operator/2
  Logical Operator/1 -> "Autonomen Modus erst wieder aktivieren, wenn jemand am Auto mit Button bestätigt oder Jetson ueber UART bescheid gibt"/2
  Logical Operator1/1 -> "Autonomen Modus erst wieder aktivieren, wenn jemand am Auto mit Button bestätigt oder Jetson ueber UART bescheid gibt"/1
  Befehl vom Jetson ueber UART Autonommodus deaktivieren/1 -> Logical Operator/3

== system STDiscovery/Debug/Subsystem ==
  In1 : Inport
  Enable : EnablePort
  IC : InitialCondition  Value=7.5
  Safety 2.5 |<--->|12.5 : Subsystem
  UART Tx : S-Function  Priority=1  FunctionName=stm32f4_usart  Parameters=configuration,uartmodule,transfer,baudrate,inputtype,outputtype,confstr,binheaderarray,binterminatorarray,asciiheader,asciiterminator,bindatalength,packetmode,varname,sampletime,sampletimestr,blockid  SFunctionDeploymentMode=off  EnableBusSupport=off  mask(stm32f4_usart){configuration=Tx, uartmodule=3, baudrate=115200, databits=8, parity=No, stopbit=1, remaptxpin=Not used, remaprxpin=Not used, flowcontrol=None, remapctspin=Not used, remaprtspin=Not used, advanceoptions=off, rxbuffersize=512, txbuffersize=512, transfer=Blocking, packetmode=Ascii, binheader='7E 7E', binterminator='03 03', porttype_double=1, porttype_single=0, porttype_int8=1, porttype_uint8=0, porttype_int16=0, porttype_uint16=0, porttype_int32=0, porttype_uint32=0, asciiformat='SET Servo Duty cycle:%f\n', rx_asciiterminator=CRLF (0x0D 0x0A - "\r\n"), tx_asciiterminator=CRLF (0x0D 0x0A - "\r\n"), storagename=S, varname=, inputtype=[1  1], outputtype=[0], binheaderarray=[0], binterminatorarray=[0], bindatalength=0, asciiheader='SET Servo Duty cycle:%f\n\r\n', asciiterminator=[2 13 10], sampletime=0.1, sampletimestr=-1, blockid=SubsystemUARTTx, confstr=[ "dummy", "0", "*", "*", "0", "*", "*", "0", "*", "*", "0", "*", "*", "1", "4", "3", "1", "4", "1", "512", "512", "1", "3", "115200", "8", "No", "1", "None", "USART3"], lastmodule=1}
      mask prompts: uartmodule "UART Module"; baudrate "Baud rate (bps)"; databits "Data bits"; stopbit "Stop bit"; remaptxpin "Tx Pin"; remaprxpin "Rx Pin"; flowcontrol "Hardware flow control"; remapctspin "HW Flow control, CTS Pin"; remaprtspin "HW Flow control, RTS Pin"; advanceoptions "Advance options"; rxbuffersize "Rx buffer size (bytes)"; txbuffersize "Tx buffer size (bytes)"; packetmode "Packet mode"; binheader "Binary header (example: '7E 7E')"; binterminator "Binary terminator (example: '03 03')"; porttype_double "Number of data port, type DOUBLE"; porttype_single "Number of data port, type SINGLE"; porttype_int8 "Number of data port, type INT8"; porttype_uint8 "Number of data port, type UINT8"; porttype_int16 "Number of data port, type INT16"; porttype_uint16 "Number of data port, type UINT16"; porttype_int32 "Number of data port, type INT32"; porttype_uint32 "Number of data port, type UINT32"; asciiformat "Ascii format"; rx_asciiterminator "End of packet"; tx_asciiterminator "End of packet"; storagename "Buffer"; varname "Var name"; inputtype "Input data type"; outputtype "Output data type"; binheaderarray "Binary header"; binterminatorarray "Binary terminator"; bindatalength "Binary data length"; asciiheader "Ascii header (printf format)"; asciiterminator "Ascii terminator"; sampletime "Sample time (sec)"; sampletimestr "Compiled sample time (sec) in string"; confstr "Configuration string"; lastmodule "Last module selected"
      mask help:
      | Data type for Ascii format
      | %u, %i, %d, %o, %x: uint32
      | %e, %g, %f: single
      | %c: int8
      mask init:
      | stm32f4_usart_callback('init');
      mask Help: web(fullfile(waijungdocroot,'stm32f4_usart_tx.htm'), '-browser')
      mask TypeOptions configuration: Setup | Tx | Rx
      mask Callback configuration: stm32f4_usart_callback('configuration');
      mask TypeOptions uartmodule: 1 | 2 | 3 | 4 | 5 | 6
      mask Callback uartmodule: stm32f4_usart_callback('uartmodule');
      mask Callback baudrate: stm32f4_usart_callback('baudrate');
      mask TypeOptions databits: 8
      mask TypeOptions parity: No | Odd | Even
      mask TypeOptions stopbit: 0.5 | 1 | 1.5 | 2
      mask TypeOptions remaptxpin: Not used | A9 | B6
      mask TypeOptions remaprxpin: Not used | A10 | B7
      mask TypeOptions flowcontrol: None | RTS | CTS | RTS/CTS
      mask Callback flowcontrol: stm32f4_usart_callback('flowcontrol');
      mask TypeOptions remapctspin: Not used | A11
      mask TypeOptions remaprtspin: Not used | A12
      mask Callback advanceoptions: stm32f4_usart_callback('advanceoptions');
      mask TypeOptions rxbuffersize: 16 | 32 | 64 | 128 | 256 | 512 | 1024 | 2048
      mask TypeOptions txbuffersize: 16 | 32 | 64 | 128 | 256 | 512 | 1024 | 2048
      mask TypeOptions transfer: Blocking | Non-Blocking
      mask Callback transfer: stm32f4_usart_callback('transfer');
      mask TypeOptions packetmode: Ascii | Binary | String Buffer
      mask Callback packetmode: stm32f4_usart_callback('packetmode');
      mask Callback binheader: stm32f4_usart_callback('binheader');
      mask Callback binterminator: stm32f4_usart_callback('binterminator');
      mask Callback porttype_double: stm32f4_usart_callback('porttype');
      mask Callback porttype_single: stm32f4_usart_callback('porttype');
      mask Callback porttype_int8: stm32f4_usart_callback('porttype');
      mask Callback porttype_uint8: stm32f4_usart_callback('porttype');
      mask Callback porttype_int16: stm32f4_usart_callback('porttype');
      mask Callback porttype_uint16: stm32f4_usart_callback('porttype');
      mask Callback porttype_int32: stm32f4_usart_callback('porttype');
      mask Callback porttype_uint32: stm32f4_usart_callback('porttype');
      mask Callback asciiformat: stm32f4_usart_callback('asciiformat');
      mask TypeOptions rx_asciiterminator: CR (0x0D - "\r") | LF (0x0A - "\n") | CRLF (0x0D 0x0A - "\r\n")
      mask Callback rx_asciiterminator: stm32f4_usart_callback('rx_asciiterminator');
      mask TypeOptions tx_asciiterminator: CR (0x0D - "\r") | LF (0x0A - "\n") | CRLF (0x0D 0x0A - "\r\n") | None
      mask Callback tx_asciiterminator: stm32f4_usart_callback('tx_asciiterminator');
      mask TypeOptions storagename: <Please insert a storage name> | S
      mask Callback storagename: stm32f4_usart_callback('storagename');
      mask Callback varname: stm32f4_usart_callback('varname');
      mask Callback sampletime: stm32f4_usart_callback('sampletime');
      mask Callback sampletimestr: stm32f4_usart_callback('sampletimestr');
      mask Callback blockid: stm32f4_usart_callback('blockid');
      mask Display: text(0.95, 0.5, 'Module: USART3_Tx\nPacket: Ascii\nTransfer: Blocking\nTs (sec): -1','ver','middle','hor','right'); port_label('input', 1,'single');
  Out1 : Outport
  wires:
  In1/1 -> IC/1
  Safety 2.5 |<--->|12.5/1(Out1) -> Out1/1, UART Tx/1
  IC/1 -> Safety 2.5 |<--->|12.5/1(In1)

== system STDiscovery/Debug/Subsystem1 ==
  In1 : Inport
  Enable : EnablePort
  IC : InitialCondition  Value=7.5
  Safety 2.5 |<--->|12.5 : Subsystem
  UART Tx1 : S-Function  Priority=1  FunctionName=stm32f4_usart  Parameters=configuration,uartmodule,transfer,baudrate,inputtype,outputtype,confstr,binheaderarray,binterminatorarray,asciiheader,asciiterminator,bindatalength,packetmode,varname,sampletime,sampletimestr,blockid  SFunctionDeploymentMode=off  EnableBusSupport=off  mask(stm32f4_usart){configuration=Tx, uartmodule=3, baudrate=115200, databits=8, parity=No, stopbit=1, remaptxpin=Not used, remaprxpin=Not used, flowcontrol=None, remapctspin=Not used, remaprtspin=Not used, advanceoptions=off, rxbuffersize=512, txbuffersize=512, transfer=Blocking, packetmode=Ascii, binheader='7E 7E', binterminator='03 03', porttype_double=1, porttype_single=0, porttype_int8=1, porttype_uint8=0, porttype_int16=0, porttype_uint16=0, porttype_int32=0, porttype_uint32=0, asciiformat='SET Motor Duty cycle:%f\n', rx_asciiterminator=CRLF (0x0D 0x0A - "\r\n"), tx_asciiterminator=CRLF (0x0D 0x0A - "\r\n"), storagename=S, varname=, inputtype=[1  1], outputtype=[0], binheaderarray=[0], binterminatorarray=[0], bindatalength=0, asciiheader='SET Motor Duty cycle:%f\n\r\n', asciiterminator=[2 13 10], sampletime=0.1, sampletimestr=-1, blockid=Subsystem1UARTTx1, confstr=[ "dummy", "0", "*", "*", "0", "*", "*", "0", "*", "*", "0", "*", "*", "1", "4", "3", "1", "4", "1", "512", "512", "1", "3", "115200", "8", "No", "1", "None", "USART3"], lastmodule=1}
      mask prompts: uartmodule "UART Module"; baudrate "Baud rate (bps)"; databits "Data bits"; stopbit "Stop bit"; remaptxpin "Tx Pin"; remaprxpin "Rx Pin"; flowcontrol "Hardware flow control"; remapctspin "HW Flow control, CTS Pin"; remaprtspin "HW Flow control, RTS Pin"; advanceoptions "Advance options"; rxbuffersize "Rx buffer size (bytes)"; txbuffersize "Tx buffer size (bytes)"; packetmode "Packet mode"; binheader "Binary header (example: '7E 7E')"; binterminator "Binary terminator (example: '03 03')"; porttype_double "Number of data port, type DOUBLE"; porttype_single "Number of data port, type SINGLE"; porttype_int8 "Number of data port, type INT8"; porttype_uint8 "Number of data port, type UINT8"; porttype_int16 "Number of data port, type INT16"; porttype_uint16 "Number of data port, type UINT16"; porttype_int32 "Number of data port, type INT32"; porttype_uint32 "Number of data port, type UINT32"; asciiformat "Ascii format"; rx_asciiterminator "End of packet"; tx_asciiterminator "End of packet"; storagename "Buffer"; varname "Var name"; inputtype "Input data type"; outputtype "Output data type"; binheaderarray "Binary header"; binterminatorarray "Binary terminator"; bindatalength "Binary data length"; asciiheader "Ascii header (printf format)"; asciiterminator "Ascii terminator"; sampletime "Sample time (sec)"; sampletimestr "Compiled sample time (sec) in string"; confstr "Configuration string"; lastmodule "Last module selected"
      mask help:
      | Data type for Ascii format
      | %u, %i, %d, %o, %x: uint32
      | %e, %g, %f: single
      | %c: int8
      mask init:
      | stm32f4_usart_callback('init');
      mask Help: web(fullfile(waijungdocroot,'stm32f4_usart_tx.htm'), '-browser')
      mask TypeOptions configuration: Setup | Tx | Rx
      mask Callback configuration: stm32f4_usart_callback('configuration');
      mask TypeOptions uartmodule: 1 | 2 | 3 | 4 | 5 | 6
      mask Callback uartmodule: stm32f4_usart_callback('uartmodule');
      mask Callback baudrate: stm32f4_usart_callback('baudrate');
      mask TypeOptions databits: 8
      mask TypeOptions parity: No | Odd | Even
      mask TypeOptions stopbit: 0.5 | 1 | 1.5 | 2
      mask TypeOptions remaptxpin: Not used | A9 | B6
      mask TypeOptions remaprxpin: Not used | A10 | B7
      mask TypeOptions flowcontrol: None | RTS | CTS | RTS/CTS
      mask Callback flowcontrol: stm32f4_usart_callback('flowcontrol');
      mask TypeOptions remapctspin: Not used | A11
      mask TypeOptions remaprtspin: Not used | A12
      mask Callback advanceoptions: stm32f4_usart_callback('advanceoptions');
      mask TypeOptions rxbuffersize: 16 | 32 | 64 | 128 | 256 | 512 | 1024 | 2048
      mask TypeOptions txbuffersize: 16 | 32 | 64 | 128 | 256 | 512 | 1024 | 2048
      mask TypeOptions transfer: Blocking | Non-Blocking
      mask Callback transfer: stm32f4_usart_callback('transfer');
      mask TypeOptions packetmode: Ascii | Binary | String Buffer
      mask Callback packetmode: stm32f4_usart_callback('packetmode');
      mask Callback binheader: stm32f4_usart_callback('binheader');
      mask Callback binterminator: stm32f4_usart_callback('binterminator');
      mask Callback porttype_double: stm32f4_usart_callback('porttype');
      mask Callback porttype_single: stm32f4_usart_callback('porttype');
      mask Callback porttype_int8: stm32f4_usart_callback('porttype');
      mask Callback porttype_uint8: stm32f4_usart_callback('porttype');
      mask Callback porttype_int16: stm32f4_usart_callback('porttype');
      mask Callback porttype_uint16: stm32f4_usart_callback('porttype');
      mask Callback porttype_int32: stm32f4_usart_callback('porttype');
      mask Callback porttype_uint32: stm32f4_usart_callback('porttype');
      mask Callback asciiformat: stm32f4_usart_callback('asciiformat');
      mask TypeOptions rx_asciiterminator: CR (0x0D - "\r") | LF (0x0A - "\n") | CRLF (0x0D 0x0A - "\r\n")
      mask Callback rx_asciiterminator: stm32f4_usart_callback('rx_asciiterminator');
      mask TypeOptions tx_asciiterminator: CR (0x0D - "\r") | LF (0x0A - "\n") | CRLF (0x0D 0x0A - "\r\n") | None
      mask Callback tx_asciiterminator: stm32f4_usart_callback('tx_asciiterminator');
      mask TypeOptions storagename: <Please insert a storage name> | S
      mask Callback storagename: stm32f4_usart_callback('storagename');
      mask Callback varname: stm32f4_usart_callback('varname');
      mask Callback sampletime: stm32f4_usart_callback('sampletime');
      mask Callback sampletimestr: stm32f4_usart_callback('sampletimestr');
      mask Callback blockid: stm32f4_usart_callback('blockid');
      mask Display: text(0.95, 0.5, 'Module: USART3_Tx\nPacket: Ascii\nTransfer: Blocking\nTs (sec): -1','ver','middle','hor','right'); port_label('input', 1,'single');
  Out1 : Outport
  wires:
  In1/1 -> IC/1
  Safety 2.5 |<--->|12.5/1(Out1) -> Out1/1, UART Tx1/1
  IC/1 -> Safety 2.5 |<--->|12.5/1(In1)

== system STDiscovery/Debug/Subsystem2 ==
  In1 : Inport
  In2 : Inport  Port=2
  In3 : Inport  Port=3
  Enable : EnablePort
  Data Type Conversion : DataTypeConversion
  Data Type Conversion1 : DataTypeConversion
  Data Type Conversion2 : DataTypeConversion
  UART Tx : S-Function  Priority=1  FunctionName=stm32f4_usart  Parameters=configuration,uartmodule,transfer,baudrate,inputtype,outputtype,confstr,binheaderarray,binterminatorarray,asciiheader,asciiterminator,bindatalength,packetmode,varname,sampletime,sampletimestr,blockid  SFunctionDeploymentMode=off  EnableBusSupport=off  mask(stm32f4_usart){configuration=Tx, uartmodule=3, baudrate=115200, databits=8, parity=No, stopbit=1, remaptxpin=Not used, remaprxpin=Not used, flowcontrol=None, remapctspin=Not used, remaprtspin=Not used, advanceoptions=off, rxbuffersize=512, txbuffersize=512, transfer=Blocking, packetmode=Ascii, binheader='7E 7E', binterminator='03 03', porttype_double=1, porttype_single=0, porttype_int8=1, porttype_uint8=0, porttype_int16=0, porttype_uint16=0, porttype_int32=0, porttype_uint32=0, asciiformat='READ Servo:%f sec, %f Prozent, %f Hz\n', rx_asciiterminator=CRLF (0x0D 0x0A - "\r\n"), tx_asciiterminator=CRLF (0x0D 0x0A - "\r\n"), storagename=S, varname=, inputtype=[3  1 1 1], outputtype=[0], binheaderarray=[0], binterminatorarray=[0], bindatalength=0, asciiheader='READ Servo:%f sec, %f Prozent, %f Hz\n\r\n', asciiterminator=[2 13 10], sampletime=0.1, sampletimestr=-1, blockid=DebugSubsystem2UARTTx, confstr=[ "dummy", "0", "*", "*", "0", "*", "*", "0", "*", "*", "0", "*", "*", "1", "4", "3", "1", "4", "1", "512", "512", "1", "3", "115200", "8", "No", "1", "None", "USART3"], lastmodule=1}
      mask prompts: uartmodule "UART Module"; baudrate "Baud rate (bps)"; databits "Data bits"; stopbit "Stop bit"; remaptxpin "Tx Pin"; remaprxpin "Rx Pin"; flowcontrol "Hardware flow control"; remapctspin "HW Flow control, CTS Pin"; remaprtspin "HW Flow control, RTS Pin"; advanceoptions "Advance options"; rxbuffersize "Rx buffer size (bytes)"; txbuffersize "Tx buffer size (bytes)"; packetmode "Packet mode"; binheader "Binary header (example: '7E 7E')"; binterminator "Binary terminator (example: '03 03')"; porttype_double "Number of data port, type DOUBLE"; porttype_single "Number of data port, type SINGLE"; porttype_int8 "Number of data port, type INT8"; porttype_uint8 "Number of data port, type UINT8"; porttype_int16 "Number of data port, type INT16"; porttype_uint16 "Number of data port, type UINT16"; porttype_int32 "Number of data port, type INT32"; porttype_uint32 "Number of data port, type UINT32"; asciiformat "Ascii format"; rx_asciiterminator "End of packet"; tx_asciiterminator "End of packet"; storagename "Buffer"; varname "Var name"; inputtype "Input data type"; outputtype "Output data type"; binheaderarray "Binary header"; binterminatorarray "Binary terminator"; bindatalength "Binary data length"; asciiheader "Ascii header (printf format)"; asciiterminator "Ascii terminator"; sampletime "Sample time (sec)"; sampletimestr "Compiled sample time (sec) in string"; confstr "Configuration string"; lastmodule "Last module selected"
      mask help:
      | Data type for Ascii format
      | %u, %i, %d, %o, %x: uint32
      | %e, %g, %f: single
      | %c: int8
      mask init:
      | stm32f4_usart_callback('init');
      mask Help: web(fullfile(waijungdocroot,'stm32f4_usart_tx.htm'), '-browser')
      mask TypeOptions configuration: Setup | Tx | Rx
      mask Callback configuration: stm32f4_usart_callback('configuration');
      mask TypeOptions uartmodule: 1 | 2 | 3 | 4 | 5 | 6
      mask Callback uartmodule: stm32f4_usart_callback('uartmodule');
      mask Callback baudrate: stm32f4_usart_callback('baudrate');
      mask TypeOptions databits: 8
      mask TypeOptions parity: No | Odd | Even
      mask TypeOptions stopbit: 0.5 | 1 | 1.5 | 2
      mask TypeOptions remaptxpin: Not used | A9 | B6
      mask TypeOptions remaprxpin: Not used | A10 | B7
      mask TypeOptions flowcontrol: None | RTS | CTS | RTS/CTS
      mask Callback flowcontrol: stm32f4_usart_callback('flowcontrol');
      mask TypeOptions remapctspin: Not used | A11
      mask TypeOptions remaprtspin: Not used | A12
      mask Callback advanceoptions: stm32f4_usart_callback('advanceoptions');
      mask TypeOptions rxbuffersize: 16 | 32 | 64 | 128 | 256 | 512 | 1024 | 2048
      mask TypeOptions txbuffersize: 16 | 32 | 64 | 128 | 256 | 512 | 1024 | 2048
      mask TypeOptions transfer: Blocking | Non-Blocking
      mask Callback transfer: stm32f4_usart_callback('transfer');
      mask TypeOptions packetmode: Ascii | Binary | String Buffer
      mask Callback packetmode: stm32f4_usart_callback('packetmode');
      mask Callback binheader: stm32f4_usart_callback('binheader');
      mask Callback binterminator: stm32f4_usart_callback('binterminator');
      mask Callback porttype_double: stm32f4_usart_callback('porttype');
      mask Callback porttype_single: stm32f4_usart_callback('porttype');
      mask Callback porttype_int8: stm32f4_usart_callback('porttype');
      mask Callback porttype_uint8: stm32f4_usart_callback('porttype');
      mask Callback porttype_int16: stm32f4_usart_callback('porttype');
      mask Callback porttype_uint16: stm32f4_usart_callback('porttype');
      mask Callback porttype_int32: stm32f4_usart_callback('porttype');
      mask Callback porttype_uint32: stm32f4_usart_callback('porttype');
      mask Callback asciiformat: stm32f4_usart_callback('asciiformat');
      mask TypeOptions rx_asciiterminator: CR (0x0D - "\r") | LF (0x0A - "\n") | CRLF (0x0D 0x0A - "\r\n")
      mask Callback rx_asciiterminator: stm32f4_usart_callback('rx_asciiterminator');
      mask TypeOptions tx_asciiterminator: CR (0x0D - "\r") | LF (0x0A - "\n") | CRLF (0x0D 0x0A - "\r\n") | None
      mask Callback tx_asciiterminator: stm32f4_usart_callback('tx_asciiterminator');
      mask TypeOptions storagename: <Please insert a storage name> | S
      mask Callback storagename: stm32f4_usart_callback('storagename');
      mask Callback varname: stm32f4_usart_callback('varname');
      mask Callback sampletime: stm32f4_usart_callback('sampletime');
      mask Callback sampletimestr: stm32f4_usart_callback('sampletimestr');
      mask Callback blockid: stm32f4_usart_callback('blockid');
      mask Display: text(0.95, 0.5, 'Module: USART3_Tx\nPacket: Ascii\nTransfer: Blocking\nTs (sec): -1','ver','middle','hor','right'); port_label('input', 1,'single'); port_label('input', 2,'single'); port_label('input', 3,'single');
  wires:
  Data Type Conversion/1 -> UART Tx/1
  In1/1 -> Data Type Conversion/1
  In3/1 -> Data Type Conversion2/1
  In2/1 -> Data Type Conversion1/1
  Data Type Conversion1/1 -> UART Tx/2
  Data Type Conversion2/1 -> UART Tx/3
